simulink model "multi_agent_setup"  (R2016a)
settings: Solver=VariableStepAuto  StartTime=0.0  StopTime=400  RelTol=1e-3
model workspace (MAT data in the model file):
  agent_signal = Simulink.Signal
  agent_signal.DataType = 'double'
  agent_signal.Dimensions = 2
  agent_signal.DimensionsMode = 'Variable'
  agent_signal.Complexity = 'real'
  agent_signal.SampleTime = -1
  agent_signal.SamplingMode = 'auto'
libraries: simulink x3, vrlib x3
settings Model: Creator=jcfinnerup  LastModifiedBy=jcfinnerup

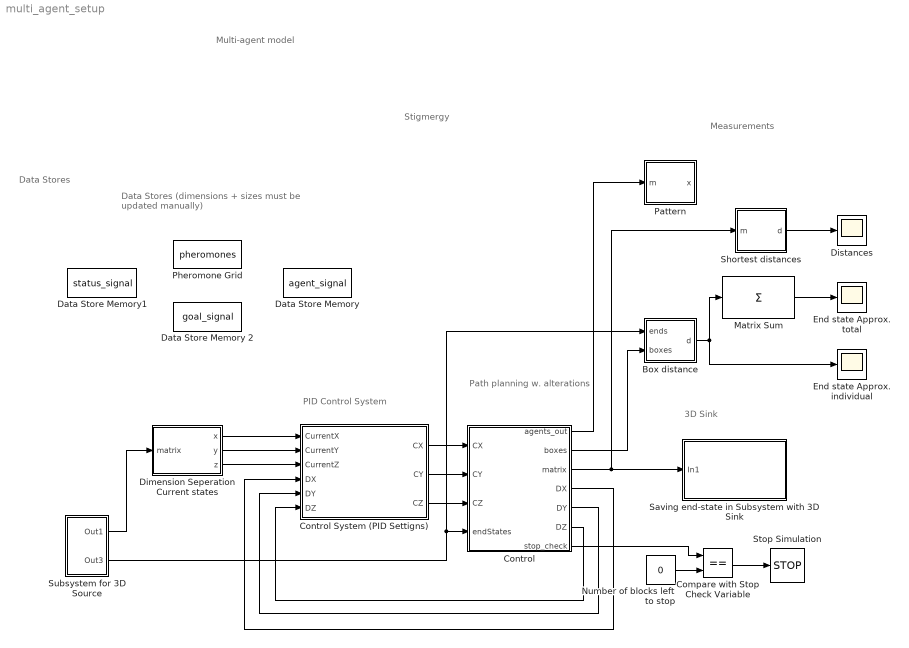
== system multi_agent_setup ==
  note: Data Stores
  note: Path planning
      | w.
      | alterations
  note: Multi-agent model
  note: PID Control System
  note: Data Stores
      | (dimensions + sizes
      | must be updated manually)
  note: 3D Sink
  note: Measurements
  note: Stigmergy
  Box distance : MATLAB Function  TreatAsAtomicUnit=on
  Compare with Stop Check Variable : RelationalOperator  Operator===  OutDataTypeStr=boolean
  Control : MATLAB Function
  Control System (PID Settigns) : Subsystem
  Data Store Memory : DataStoreMemory  DataStoreName=agent_signal  ReadBeforeWriteMsg=warning  WriteAfterWriteMsg=warning  WriteAfterReadMsg=warning  InitialValue=zeros(5, 6)  VectorParams1D=off  ShowAdditionalParam=off  OutDataTypeStr=double
  Data Store Memory 2 : DataStoreMemory  DataStoreName=goal_signal  ReadBeforeWriteMsg=warning  WriteAfterWriteMsg=warning  WriteAfterReadMsg=warning  InitialValue=[0, 0, 0, 0, 0, 0, 0, 0, 0]  VectorParams1D=off  ShowAdditionalParam=off  OutDataTypeStr=double
  Data Store Memory1 : DataStoreMemory  DataStoreName=status_signal  ReadBeforeWriteMsg=warning  WriteAfterWriteMsg=warning  WriteAfterReadMsg=warning  InitialValue=zeros(9,1)  VectorParams1D=off  ShowAdditionalParam=off  OutDataTypeStr=double
  "Dimension Seperation Current states " : MATLAB Function  TreatAsAtomicUnit=on
  Distances : Scope
  End state Approx. individual : Scope
  End state Approx. total : Scope
  Matrix Sum : Sum  Inputs=+
  Number of blocks left to stop : Constant  Value=0
  Pattern : MATLAB Function  TreatAsAtomicUnit=on
  Pheromone Grid : DataStoreMemory  DataStoreName=pheromones  ReadBeforeWriteMsg=warning  WriteAfterWriteMsg=warning  WriteAfterReadMsg=warning  InitialValue=zeros(30, 10, 10)  VectorParams1D=off  ShowAdditionalParam=off  OutDataTypeStr=double
  Saving end-state in Subsystem with 3D Sink : Subsystem
  Shortest distances : MATLAB Function  TreatAsAtomicUnit=on
  Stop Simulation : Stop
  Subsystem for 3D Source : Subsystem
  wires:
  "Dimension Seperation Current states "/1(x) -> Control System (PID Settigns)/1(CurrentX)
  "Dimension Seperation Current states "/2(y) -> Control System (PID Settigns)/2(CurrentY)
  "Dimension Seperation Current states "/3(z) -> Control System (PID Settigns)/3(CurrentZ)
  Control System (PID Settigns)/2(CY) -> Control/2(CY)
  Control System (PID Settigns)/3(CZ) -> Control/3(CZ)
  Control System (PID Settigns)/1(CX) -> Control/1(CX)
  Control/4(DX) -> Control System (PID Settigns)/4(DX)
  Control/5(DY) -> Control System (PID Settigns)/5(DY)
  Control/6(DZ) -> Control System (PID Settigns)/6(DZ)
  Number of blocks left to stop/1 -> Compare with Stop Check Variable/2
  Control/7(stop_check) -> Compare with Stop Check Variable/1
  Compare with Stop Check Variable/1 -> Stop Simulation/1
  Box distance/1(d) -> End state Approx. individual/1, Matrix Sum/1
  Matrix Sum/1 -> End state Approx. total/1
  Control/3(matrix) -> Shortest distances/1(m), Saving end-state in Subsystem with 3D Sink/1(In1)
  Subsystem for 3D Source/2(Out3) -> Box distance/1(ends), Control/4(endStates)
  Subsystem for 3D Source/1(Out1) -> "Dimension Seperation Current states "/1(matrix)
  Shortest distances/1(d) -> Distances/1
  Control/2(boxes) -> Box distance/2(boxes)
  Control/1(agents_out) -> Pattern/1(m)

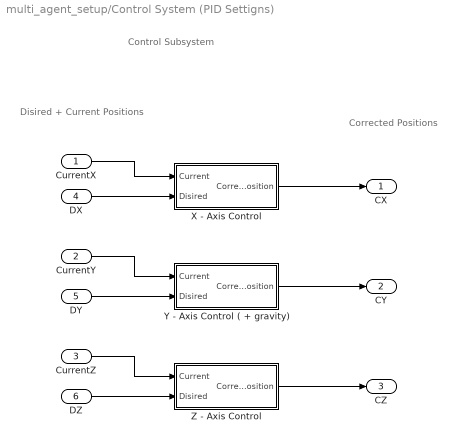
== system multi_agent_setup/Control System (PID Settigns) ==
  note: Control Subsystem
  note: Corrected
      | Positions
  note: Disired + Current
      | Positions
  CurrentX : Inport
  CurrentY : Inport  Port=2
  CurrentZ : Inport  Port=3
  DX : Inport  Port=4
  DY : Inport  Port=5
  DZ : Inport  Port=6
  X - Axis Control : Subsystem
  Y - Axis Control ( + gravity) : Subsystem
  Z - Axis Control : Subsystem
  CX : Outport
  CY : Outport  Port=2
  CZ : Outport  Port=3
  wires:
  CurrentX/1 -> X - Axis Control/1(Current)
  DX/1 -> X - Axis Control/2(Disired)
  DY/1 -> Y - Axis Control ( + gravity)/2(Disired)
  CurrentY/1 -> Y - Axis Control ( + gravity)/1(Current)
  DZ/1 -> Z - Axis Control/2(Disired)
  CurrentZ/1 -> Z - Axis Control/1(Current)
  X - Axis Control/1(Corrected Position) -> CX/1
  Y - Axis Control ( + gravity)/1(Corrected Position) -> CY/1
  Z - Axis Control/1(Corrected Position) -> CZ/1

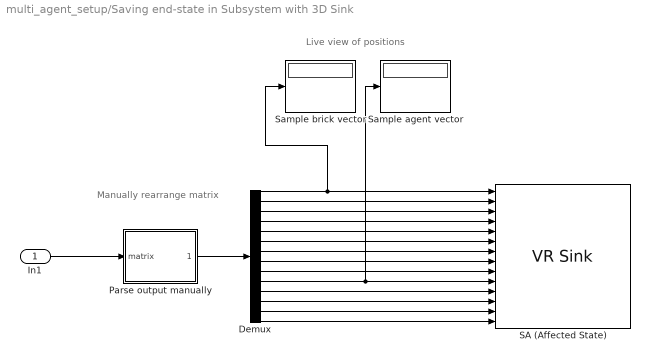
== system multi_agent_setup/Saving end-state in Subsystem with 3D Sink ==
  note: Manually rearrange
      | matrix
  note: Live view of positions
  In1 : Inport
  Demux : Demux  Outputs=14
  Parse output manually : MATLAB Function  TreatAsAtomicUnit=on
  "SA (Affected State) " : vrlib/VR Sink  InstantiateOnLoad=on  SampleTime=0.1  ViewEnable=on  RemoteChange=off  RemoteView=off  FieldsWritten=B1.translation.3.1.1.double#B2.translation.3.1.1.double#B3.translation.3.1.1.double#B4.translation.3.1.1.double#B5.translation.3.1.1.double#B6.translation.3.1.1.double#B7.translation.3.1.1.double#B8.translation.3.1.1.double#B9.translation.3.1.1.double#A1.translation.3.1.1.double#A2.translation.3.1.1.double#A3.translation.3.1.1.double#A4.translation.3.1.1.double#A5.translation.3.1.1.double  WorldFileName=VR3D_MA/multi_agent_setup.wrl  WorldDescription=Multi Agent Track  AutoView=off  VideoDimensions=[]  AllowVariableSize=off
  Sample agent vector : Display
  "Sample brick vector " : Display
  wires:
  In1/1 -> Parse output manually/1(matrix)
  Demux/10 -> Sample agent vector/1, "SA (Affected State) "/10
  Demux/1 -> "Sample brick vector "/1, "SA (Affected State) "/1
  Parse output manually/1(formatted) -> Demux/1
  Demux/2 -> "SA (Affected State) "/2
  Demux/3 -> "SA (Affected State) "/3
  Demux/4 -> "SA (Affected State) "/4
  Demux/5 -> "SA (Affected State) "/5
  Demux/6 -> "SA (Affected State) "/6
  Demux/7 -> "SA (Affected State) "/7
  Demux/8 -> "SA (Affected State) "/8
  Demux/9 -> "SA (Affected State) "/9
  Demux/11 -> "SA (Affected State) "/11
  Demux/13 -> "SA (Affected State) "/13
  Demux/12 -> "SA (Affected State) "/12
  Demux/14 -> "SA (Affected State) "/14

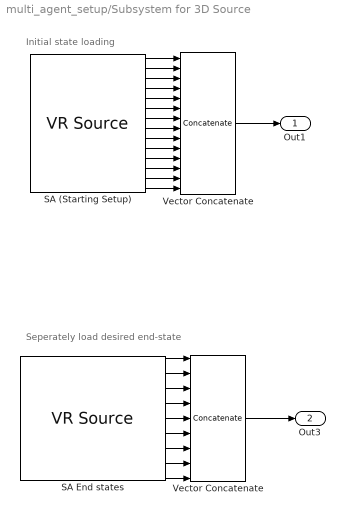
== system multi_agent_setup/Subsystem for 3D Source ==
  note: Initial state loading
  note: Seperately load desired end-state
  "SA End states " : vrlib/VR Source  InstantiateOnLoad=on  SampleTime=0.1  ViewEnable=on  RemoteChange=off  RemoteView=off  FieldsRead=E1.translation.1.3.1.double#E2.translation.1.3.1.double#E3.translation.1.3.1.double#E4.translation.1.3.1.double#E5.translation.1.3.1.double#E6.translation.1.3.1.double#E7.translation.1.3.1.double#E8.translation.1.3.1.double#E9.translation.1.3.1.double  WorldFileName=VR3D_MA/multi_agent_setup.wrl  WorldDescription=Single Agent Track  AutoView=off  VideoDimensions=[]  AllowVariableSize=off
  SA (Starting Setup) : vrlib/VR Source  InstantiateOnLoad=on  SampleTime=1  ViewEnable=on  RemoteChange=off  RemoteView=off  FieldsRead=B1.translation.1.3.1.double#B2.translation.1.3.1.double#B3.translation.1.3.1.double#B4.translation.1.3.1.double#B5.translation.1.3.1.double#B6.translation.1.3.1.double#B7.translation.1.3.1.double#B8.translation.1.3.1.double#B9.translation.1.3.1.double#A1.translation.1.3.1.double#A2.translation.1.3.1.double#A3.translation.1.3.1.double#A4.translation.1.3.1.double#A5.translation.1.3.1.double  WorldFileName=VR3D_MA/multi_agent_setup.wrl  WorldDescription=Multi Agent Track  AutoView=off  VideoDimensions=[]  AllowVariableSize=off  FigureProperties="{'Position', 'Name', 'Viewpoint', 'CameraBound', 'CameraDirection', 'CameraPosition', 'CameraUpVector', 'ZoomFactor', 'Antialiasing', 'Headlight', 'Lighting', 'NavPanel', 'Sound', 'StatusBar', 'Stereo3D', 'Stereo3DCameraOffset', 'Stereo3DHIT', 'ToolBar', 'Textures', 'Transparency', 'Triad', 'Wireframe', 'NavZones', 'NavMode', 'NavSpeed', 'CaptureFileFormat', 'CaptureFileName', 'Record2DCompressMethod', 'Record2DCompressQuality', 'Record2D', 'Record2DFileName', 'Record2DFPS'; [5.0000000000000000e+00   9.5000000000000000e+01   7.6400000000000000e+02   3.9400000000000000e+02], 'Single Agent Track', '_untitled_1', 'on', [-6.2790506997431925e-02   0.0000000000000000e+00  -9.9802672921671065e-01], [-3.1410752802896701e-02   0.0000000000000000e+00  -1.9995065605629385e+00], [0.0000000000000000e+00   1.0000000000000000e+00   0.0000000000000000e+00], [1.0000000000000000e+00], 'on', 'on', 'on', 'halfbar', 'on', 'on', 'off', [1.0000000149011612e-01], [0.0000000000000000e+00], 'on', 'on', 'on', 'none', 'off', 'off', 'fly', 'normal', 'tif', '%f_anim_%n.tif', 'auto', [7.5000000000000000e+01], 'off', '%f_anim_%n.avi', 'auto'}"
  Vector Concatenate : Concatenate  NumInputs=14  Mode=Multidimensional array  ConcatenateDimension=2
  "Vector Concatenate " : Concatenate  NumInputs=9  Mode=Multidimensional array  ConcatenateDimension=2
  Out1 : Outport
  Out3 : Outport  Port=2
  wires:
  Vector Concatenate/1 -> Out1/1
  "Vector Concatenate "/1 -> Out3/1
  "SA End states "/1 -> "Vector Concatenate "/1
  "SA End states "/2 -> "Vector Concatenate "/2
  "SA End states "/3 -> "Vector Concatenate "/3
  "SA End states "/4 -> "Vector Concatenate "/4
  "SA End states "/5 -> "Vector Concatenate "/5
  "SA End states "/6 -> "Vector Concatenate "/6
  "SA End states "/7 -> "Vector Concatenate "/7
  "SA End states "/8 -> "Vector Concatenate "/8
  "SA End states "/9 -> "Vector Concatenate "/9
  SA (Starting Setup)/1 -> Vector Concatenate/1
  SA (Starting Setup)/2 -> Vector Concatenate/2
  SA (Starting Setup)/3 -> Vector Concatenate/3
  SA (Starting Setup)/4 -> Vector Concatenate/4
  SA (Starting Setup)/5 -> Vector Concatenate/5
  SA (Starting Setup)/6 -> Vector Concatenate/6
  SA (Starting Setup)/7 -> Vector Concatenate/7
  SA (Starting Setup)/8 -> Vector Concatenate/8
  SA (Starting Setup)/9 -> Vector Concatenate/9
  SA (Starting Setup)/10 -> Vector Concatenate/10
  SA (Starting Setup)/11 -> Vector Concatenate/11
  SA (Starting Setup)/12 -> Vector Concatenate/12
  SA (Starting Setup)/13 -> Vector Concatenate/13
  SA (Starting Setup)/14 -> Vector Concatenate/14

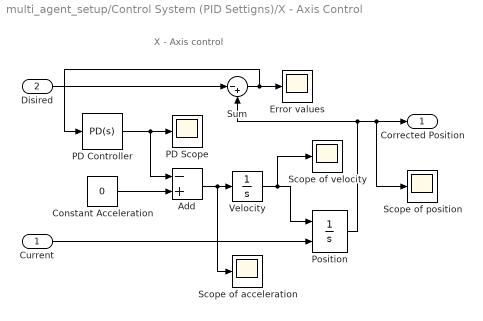
== system multi_agent_setup/Control System (PID Settigns)/X - Axis Control ==
  note: X - Axis control
  Current : Inport
  Disired : Inport  Port=2
  Add : Sum  Inputs=-+  OutMin=-5  OutMax=5
  Constant Acceleration : Constant  Value=0
  Error values : Scope
  PD Controller : simulink/Continuous/PID Controller  Controller=PD  TimeDomain=Continuous-time  SampleTime=-1  IntegratorMethod=Forward Euler  FilterMethod=Forward Euler  Form=Ideal  UseFilter=on  ControllerParametersSource=internal  P=1.6  I=5  D=1.8  N=100  InitialConditionSource=internal  InitialConditionForIntegrator=10  InitialConditionForFilter=0  ExternalReset=none  LimitOutput=on  UpperSaturationLimit=20  LowerSaturationLimit=-20  LinearizeAsGain=off  AntiWindupMode=none  Kb=1  TrackingMode=off  Kt=1  PParamMin=[]  PParamMax=[]  IParamMin=[]  IParamMax=[]  DParamMin=[]  DParamMax=[]  NParamMin=[]  NParamMax=[]  KbParamMin=[]  KbParamMax=[]  KtParamMin=[]  KtParamMax=[]  POutMin=[]  POutMax=[]  IOutMin=[]  IOutMax=[]  DOutMin=[]  DOutMax=[]  NOutMin=[]  NOutMax=[]  KbOutMin=[]  KbOutMax=[]  KtOutMin=[]  KtOutMax=[]  IntegratorOutMin=[]  IntegratorOutMax=[]  FilterOutMin=[]  FilterOutMax=[]  SumOutMin=[]  SumOutMax=[]  SumI1OutMin=[]  SumI1OutMax=[]  SumI2OutMin=[]  SumI2OutMax=[]  SumI3OutMin=[]  SumI3OutMax=[]  SumDOutMin=[]  SumDOutMax=[]  SaturationOutMin=[]  SaturationOutMax=[]  IntegratorContinuousStateAttributes=''  IntegratorStateMustResolveToSignalObject=off  IntegratorRTWStateStorageClass=Auto  FilterContinuousStateAttributes=''  FilterStateMustResolveToSignalObject=off  FilterRTWStateStorageClass=Auto  DifferentiatorICPrevScaledInput=0  DifferentiatorOutMin=[]  DifferentiatorOutMax=[]
  PD Scope : Scope
  Position : Integrator  InitialConditionSource=external  LowerSaturationLimit=0  ZeroCross=off
  Scope of position : Scope
  Scope of velocity : Scope
  Scope of acceleration : Scope
  Sum : Sum  Inputs=|-+
  Velocity : Integrator  LimitOutput=on  UpperSaturationLimit=15  LowerSaturationLimit=-15  ZeroCross=off
  Corrected Position : Outport
  wires:
  Disired/1 -> Sum/1
  Sum/1 -> PD Controller/1, Error values/1
  PD Controller/1 -> PD Scope/1, Add/1
  Add/1 -> Scope of acceleration/1, Velocity/1
  Current/1 -> Position/2
  Position/1 -> Sum/2, Scope of position/1, Corrected Position/1
  Velocity/1 -> Scope of velocity/1, Position/1
  Constant Acceleration/1 -> Add/2

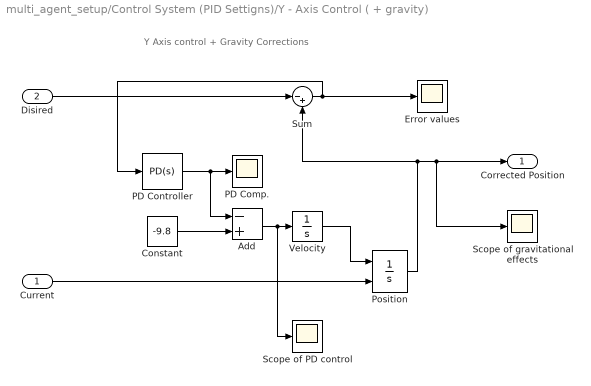
== system multi_agent_setup/Control System (PID Settigns)/Y - Axis Control ( + gravity) ==
  note: Y Axis control + Gravity Corrections
  Current : Inport
  Disired : Inport  Port=2
  Add : Sum  Inputs=-+  OutMin=[-9.8]
  Constant : Constant  Value=-9.8
  Error values : Scope
  "PD Comp. " : Scope
  PD Controller : simulink/Continuous/PID Controller  Controller=PD  TimeDomain=Continuous-time  SampleTime=-1  IntegratorMethod=Forward Euler  FilterMethod=Forward Euler  Form=Parallel  UseFilter=on  ControllerParametersSource=internal  P=5  I=1  D=2  N=100  InitialConditionSource=internal  InitialConditionForIntegrator=10  InitialConditionForFilter=0  ExternalReset=none  LimitOutput=on  UpperSaturationLimit=0  LowerSaturationLimit=-50  LinearizeAsGain=on  AntiWindupMode=none  Kb=1  TrackingMode=off  Kt=1  PParamMin=[]  PParamMax=[]  IParamMin=[]  IParamMax=[]  DParamMin=[]  DParamMax=[]  NParamMin=[]  NParamMax=[]  KbParamMin=[]  KbParamMax=[]  KtParamMin=[]  KtParamMax=[]  POutMin=[]  POutMax=[]  IOutMin=[]  IOutMax=[]  DOutMin=[]  DOutMax=[]  NOutMin=[]  NOutMax=[]  KbOutMin=[]  KbOutMax=[]  KtOutMin=[]  KtOutMax=[]  IntegratorOutMin=[]  IntegratorOutMax=[]  FilterOutMin=[]  FilterOutMax=[]  SumOutMin=[]  SumOutMax=[]  SumI1OutMin=[]  SumI1OutMax=[]  SumI2OutMin=[]  SumI2OutMax=[]  SumI3OutMin=[]  SumI3OutMax=[]  SumDOutMin=[]  SumDOutMax=[]  SaturationOutMin=[]  SaturationOutMax=[]  IntegratorContinuousStateAttributes=''  IntegratorStateMustResolveToSignalObject=off  IntegratorRTWStateStorageClass=Auto  FilterContinuousStateAttributes=''  FilterStateMustResolveToSignalObject=off  FilterRTWStateStorageClass=Auto  DifferentiatorICPrevScaledInput=0  DifferentiatorOutMin=[]  DifferentiatorOutMax=[]
  Position : Integrator  InitialConditionSource=external  LimitOutput=on  LowerSaturationLimit=0  ZeroCross=off
  Scope of PD control : Scope
  "Scope of gravitational effects " : Scope
  Sum : Sum  Inputs=|-+
  Velocity : Integrator  ZeroCross=off
  Corrected Position : Outport
  wires:
  Constant/1 -> Add/2
  Velocity/1 -> Position/1
  Position/1 -> Corrected Position/1, "Scope of gravitational effects "/1, Sum/2
  Current/1 -> Position/2
  Add/1 -> Scope of PD control/1, Velocity/1
  PD Controller/1 -> "PD Comp. "/1, Add/1
  Sum/1 -> PD Controller/1, Error values/1
  Disired/1 -> Sum/1

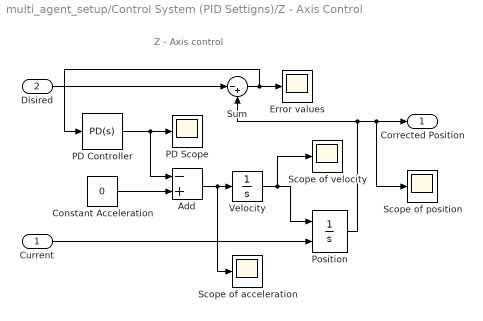
== system multi_agent_setup/Control System (PID Settigns)/Z - Axis Control ==
  note: Z - Axis control
  Current : Inport
  Disired : Inport  Port=2
  Add : Sum  Inputs=-+  OutMin=-5  OutMax=5
  Constant Acceleration : Constant  Value=0
  Error values : Scope
  PD Controller : simulink/Continuous/PID Controller  Controller=PD  TimeDomain=Continuous-time  SampleTime=-1  IntegratorMethod=Forward Euler  FilterMethod=Forward Euler  Form=Ideal  UseFilter=on  ControllerParametersSource=internal  P=1.6  I=5  D=1.8  N=100  InitialConditionSource=internal  InitialConditionForIntegrator=10  InitialConditionForFilter=0  ExternalReset=none  LimitOutput=on  UpperSaturationLimit=20  LowerSaturationLimit=-20  LinearizeAsGain=off  AntiWindupMode=none  Kb=1  TrackingMode=off  Kt=1  PParamMin=[]  PParamMax=[]  IParamMin=[]  IParamMax=[]  DParamMin=[]  DParamMax=[]  NParamMin=[]  NParamMax=[]  KbParamMin=[]  KbParamMax=[]  KtParamMin=[]  KtParamMax=[]  POutMin=[]  POutMax=[]  IOutMin=[]  IOutMax=[]  DOutMin=[]  DOutMax=[]  NOutMin=[]  NOutMax=[]  KbOutMin=[]  KbOutMax=[]  KtOutMin=[]  KtOutMax=[]  IntegratorOutMin=[]  IntegratorOutMax=[]  FilterOutMin=[]  FilterOutMax=[]  SumOutMin=[]  SumOutMax=[]  SumI1OutMin=[]  SumI1OutMax=[]  SumI2OutMin=[]  SumI2OutMax=[]  SumI3OutMin=[]  SumI3OutMax=[]  SumDOutMin=[]  SumDOutMax=[]  SaturationOutMin=[]  SaturationOutMax=[]  IntegratorContinuousStateAttributes=''  IntegratorStateMustResolveToSignalObject=off  IntegratorRTWStateStorageClass=Auto  FilterContinuousStateAttributes=''  FilterStateMustResolveToSignalObject=off  FilterRTWStateStorageClass=Auto  DifferentiatorICPrevScaledInput=0  DifferentiatorOutMin=[]  DifferentiatorOutMax=[]
  PD Scope : Scope
  Position : Integrator  InitialConditionSource=external  LowerSaturationLimit=0  ZeroCross=off
  Scope of position : Scope
  Scope of velocity : Scope
  Scope of acceleration : Scope
  Sum : Sum  Inputs=|-+
  Velocity : Integrator  LimitOutput=on  UpperSaturationLimit=15  LowerSaturationLimit=-15  ZeroCross=off
  Corrected Position : Outport
  wires:
  Disired/1 -> Sum/1
  Sum/1 -> PD Controller/1, Error values/1
  PD Controller/1 -> PD Scope/1, Add/1
  Add/1 -> Scope of acceleration/1, Velocity/1
  Current/1 -> Position/2
  Position/1 -> Sum/2, Scope of position/1, Corrected Position/1
  Velocity/1 -> Scope of velocity/1, Position/1
  Constant Acceleration/1 -> Add/2

== matlab function multi_agent_setup/Box distance ==
  data: ends input; d output; boxes input
function d = dist(ends, boxes)
%#codegen


    distance = zeros(1,length(ends));

    
    for i=1:length(ends)
        this_vec = abs(ends(:,i) - boxes(:,i));
        this_dist = norm(this_vec);
        distance(1, i) = this_dist;
    end
    
d = distance;

== matlab function multi_agent_setup/Shortest distances ==
  data: m input; d output
function d = dist(m)
%#codegen


% This function is used to calculate the shortest distance from
% the agents and blocks to other agents or blocks

    distance_threshold = 15;

    % Matrix to hold distance
    matrix = m(:,10:end);
    distance = zeros(1,length(matrix(1,:))+1);
    distance(1,end) = distance_threshold;
    
    % Compute Euclidian distance to nearest object
    for i=1:length(matrix(1,:))
        distance(1,i) = 500;
        this_pos = matrix(:,i);
        
        for j=1:length(matrix(1,:))
            % Skip if comparing with self
            if j == i
                continue;
            end
            
            % Calc 3D distance
            this_vec = abs(this_pos - matrix(:,j));
            this_dist = norm(this_vec);
            if distance(1,i) > this_dist
                distance(1,i) = this_dist;
            end
        end
    end
    
d = distance;

== matlab function multi_agent_setup/Pattern ==
  data: m input; x output
function x= top_view(m)
%#codegen


    % Matrix to hold distance
    x = m(1,:)

== matlab function multi_agent_setup/Dimension Seperation Current states  ==
  data: x output; y output; z output; matrix input

function [x,y,z] =  fun(matrix)
    x = matrix(1,:)
    y = matrix(2,:)
    z = matrix(3,:)

== matlab function multi_agent_setup/Control ==
  data: agents_out output; boxes output; CX input; CY input; CZ input; endStates input; matrix output; DX output; DY output; DZ output; agent_signal data_store_memory; status_signal data_store_memory; goal_signal data_store_memory; stop_check output; pheromones data_store_memory
function [agents_out, boxes, matrix, DX, DY, DZ, stop_check] = fcn(CX, CY, CZ, endStates)
%#codegen

    % World Constants 
    block_height = 6;
    block_width = 10;
    last_box_at = 9;
    agents_at = [10, 11, 12, 13, 14]; % Denotes the indices of the agents
    threshold = 2;
    search_height = 10;
    x_len = 300;
    y_len = 100;
    z_len = 100;
    stand_still_threshold = 2;
    agent_view_radius = 20;
        
    % Variables
    % (Status of box, status of goal)
    % 0: nothing, 1:moving, 2:completed
    global status_signal;
    blocks_moving_to = status_signal;
    
    % (Index of agent, index of end state
    global agent_signal;
    agents_moving_to = agent_signal;
    
    % Pheromones
    global pheromones;
    
    % Assign it not pre-assigned

    % Mapping Dimensions of End-States
    EX = endStates(1,:);
    EY = endStates(2,:);
    EZ = endStates(3,:);
    
    % Creating Desired Positions From Current Positions
    DX = CX;
    DY = CY;
    DZ = CZ;

    % Check if simulation is completed
    stop_check = sum(ismember(ismember(blocks_moving_to, 2),0));
    
    % Looping through Objects
    % This is the control loop where desired positions are changed
    % Nothing is changed if the agent is already on the way to 
    % the desired position
    % or if the end states are already fulfilled
    
    % Decrease the pheromones
    %pheromones = pheromones -.1;
    
    % Overwrite physics for boxes for completed goals
    for i = 1:length(blocks_moving_to)    
        if blocks_moving_to(i) == 2 % 2 for completed
            CX(i) = EX(i);
            CY(i) = EY(i);
            CZ(i) = EZ(i);
        end
    end
    
    % Assign Desired Positions
    for i = 1:length(agents_at)
        index_of_agent = agents_at(i);
        
        % Agent Positions
        agent_x = CX(index_of_agent);
        agent_y = CY(index_of_agent);
        agent_z = CZ(index_of_agent);        
        agent_pos = [agent_x agent_y agent_z];
        
        % Pheromone Index
        p_index_x = floor((agent_x/10)+16);
        p_index_y = floor((agent_y/10)+6);
        p_index_z = floor((agent_z/10)+6);
        
        if p_index_z < 1 
            p_index_z = 1;
        elseif p_index_z > 10 
            p_index_z = 10 ;
        end
        
        if p_index_y < 1 
            p_index_y = 1;
        elseif p_index_y > 10 
            p_index_y = 10 ;
        end
        
        if p_index_x < 1 
            p_index_x = 1;
        elseif p_index_x > 30 
            p_index_x = 30 ;
        end
        
        curr_p_index = [p_index_x, p_index_y, p_index_z];
        
        % Value of current pheromone
        % 0: Empty, 1: 
        cur_p_value = pheromones(p_index_x, p_index_y, p_index_z);
        
        % Setting current value to something
        % pheromones(p_index_x, p_index_y, p_index_z) = 0;


        % Assign movement towards box
        if agents_moving_to(i,1) == 0

            % Value, Index of highest element
            [maxval, maxind] = max(pheromones(:));
            [maxxidx, maxyidx, maxzidx] = ind2sub(size(pheromones),maxind);
            
            
            % Agent data
            % 1: State
            % 2,3,4: Coordinates of desired movement
            % 5: Box to carry
            % 6: Pheromoned or random (0:random, 1:p, 2:new p)
            
            if maxval == 0
                disp('Global random')
                agents_moving_to(i, 1) = 1;
                agents_moving_to(i, 2) = randi([-149 149],1,1);
                agents_moving_to(i, 3) = search_height; 
                agents_moving_to(i, 4) = randi([-49 49],1,1);
            elseif agents_moving_to(i, 6) == 0;
                disp('Global Pheromone')
                agents_moving_to(i, 1) = 1;
                agents_moving_to(i, 6) = 1;
                agents_moving_to(i, 2) = maxxidx*10-150;
                agents_moving_to(i, 3) = search_height; 
                agents_moving_to(i, 4) = maxzidx*10-50;
            else % if pheromoned
                periph = pheromones(p_index_x-1:p_index_x+1,p_index_y-1:p_index_y+1,p_index_z-1:p_index_z+1);
                periph(2,2,2) = 0;
                [maxval, maxind] = max(periph(:));
                [maxxidx, maxyidx, maxzidx] = ind2sub(size(periph),maxind);
                
                if maxval == 0 || agents_moving_to(i, 6) == 2
                    disp('Local random')
                    agents_moving_to(i, 1) = 1;
                    agents_moving_to(i, 6) = 0;
                    agents_moving_to(i, 2) = randi([agent_x-20 agent_x+20],1,1);
                    agents_moving_to(i, 3) = search_height; 
                    agents_moving_to(i, 4) = randi([agent_z-20 agent_z+20],1,1);
                else
                    disp('Local Pheromone')
                    agents_moving_to(i, 1) = 1;
                    agents_moving_to(i, 6) = 2;
                    agents_moving_to(i, 2) = maxxidx*10-150;
                    agents_moving_to(i, 3) = search_height; 
                    agents_moving_to(i, 4) = maxzidx*10-50; 
                end
            end
            
        elseif agents_moving_to(i,1) == 1
            
            DX(index_of_agent) = agents_moving_to(i, 2);
            DY(index_of_agent) = agents_moving_to(i, 3);
            DZ(index_of_agent) = agents_moving_to(i, 4);
            
            C = [CX(index_of_agent) CY(index_of_agent) CZ(index_of_agent)];

            % Boxes
            box_dist = agent_view_radius;
            closest_box_index = 0;
            for b = 1:last_box_at 
                dist = max(abs([CX(b) CY(b) CZ(b)] - C));
                if blocks_moving_to(b) == 0 && dist <= box_dist
                    box_dist = dist;
                    closest_box_index = b;
                end
            end
            
            if closest_box_index > 0
                DX(index_of_agent) = CX(closest_box_index);
                DY(index_of_agent) = CY(closest_box_index) + block_height;
                DZ(index_of_agent) = CZ(closest_box_index);
            end
                
            D = [DX(index_of_agent) DY(index_of_agent) DZ(index_of_agent)];
            
            % Check if they are standing still, reset
            if max(abs(C-D)) < stand_still_threshold
                if closest_box_index > 0
                    agents_moving_to(i, 1) = 2;
                    blocks_moving_to(closest_box_index) = 1;
                    agents_moving_to(i, 5) = closest_box_index;
                    pheromones(p_index_x, p_index_y, p_index_z) = 10;  
                elseif agents_moving_to(i, 6) == 0; % if not pheromoned
                    agents_moving_to(i, 1) = 0;
                    disp('Back to search 1');
                else
                    agents_moving_to(i, 1) = 0;
                    disp('Back to search 0');
                end
            end
                        
        
        % Assign movement towards goal
        elseif agents_moving_to(i,1) == 2
            
            % Value, Index of highest element
            [maxval, maxind] = max(pheromones(:));
            [maxxidx, maxyidx, maxzidx] = ind2sub(size(pheromones),maxind);

            if maxval == 0 
                agents_moving_to(i, 1) = 3;
                agents_moving_to(i, 2) = randi([-149 149],1,1);
                agents_moving_to(i, 3) = search_height; 
                agents_moving_to(i, 4) = randi([-49 49],1,1);
            else
                agents_moving_to(i, 1) = 3;
                agents_moving_to(i, 2) = randi([-149 149],1,1);
                agents_moving_to(i, 3) = search_height; 
                agents_moving_to(i, 4) = randi([-49 49],1,1);
            end
            
        elseif agents_moving_to(i,1) == 3
            
            
            index_of_carried = agents_moving_to(i,5);
            
            CX(index_of_carried) = CX(agents_at(i));
            CY(index_of_carried) = CY(agents_at(i))-block_height*.5;
            CZ(index_of_carried) = CZ(agents_at(i));
            
            C = [CX(index_of_agent) CY(index_of_agent) CZ(index_of_agent)];
            
            % Goals
            goal_dist = agent_view_radius;
            closest_goal_index = 0;
            for b = 1:last_box_at 
                dist = max(abs([EX(b) EY(b) EZ(b)] - C));
                if dist <= goal_dist
                    goal_dist = dist;
                    closest_goal_index = b;
                end
            end
            
            % Check if they are standing still, reset
            if closest_goal_index > 0
                DX(index_of_agent) = EX(closest_goal_index);
                DY(index_of_agent) = EY(closest_goal_index)+block_height;
                DZ(index_of_agent) = EZ(closest_goal_index);
            else
                DX(index_of_agent) = agents_moving_to(i, 2);
                DY(index_of_agent) = agents_moving_to(i, 3);
                DZ(index_of_agent) = agents_moving_to(i, 4);
            end
          
            D = [DX(index_of_agent) DY(index_of_agent) DZ(index_of_agent)];
            
            % Check if they are standing still, reset
            if max(abs(C-D)) < stand_still_threshold
                if closest_goal_index > 0
                    agents_moving_to(i, 1) = 0;
                    agents_moving_to(i, 5) = 0;
                    blocks_moving_to(index_of_carried) = 2;
                else
                    agents_moving_to(i, 1) = 2;
                end
            end
        end
    end
    
    % Update Global Variables
    agent_signal = agents_moving_to;
    status_signal = blocks_moving_to;

    matrix = [CX;CY;CZ];
    boxes = matrix(1:end,1:end-length(agents_at));
    agents_out = matrix(1:end, agents_at(1):end);

== matlab function multi_agent_setup/Saving end-state in Subsystem with 3D Sink/Parse output manually ==
  data: matrix input; formatted output
function formatted = fcn(matrix)
%#codegen

formatted = [
    matrix(:,1)
    matrix(:,2)
    matrix(:,3)
    matrix(:,4)
    matrix(:,5)
    matrix(:,6)
    matrix(:,7)
    matrix(:,8)
    matrix(:,9)
    matrix(:,10)
    matrix(:,11)
    matrix(:,12)
    matrix(:,13)
    matrix(:,14)
];
